simulink model "MRAC_PIDresp"  (R2018a)
settings: Solver=VariableStepAuto  StartTime=0.0  StopTime=100  RelTol=1e-3
values from neighbouring files (symbols this model uses):
  gam_p = 5    [MRAC_test.m]
  gam_pcmd = .1    (= 0.1)    [MRAC_test.m]
  k_d = 0.00073    [MRAC_test.m]
  k_i = 0    [MRAC_test.m]
  k_p = 0.0038    [MRAC_test.m]
  ref_den = [coef_a coef_b coef_c]    [MRAC_test.m]
  ref_num = [coef_c]    [MRAC_test.m]
libraries: simulink_extras x1
settings Model: Creator=ctf365  LastModifiedBy=ctf365

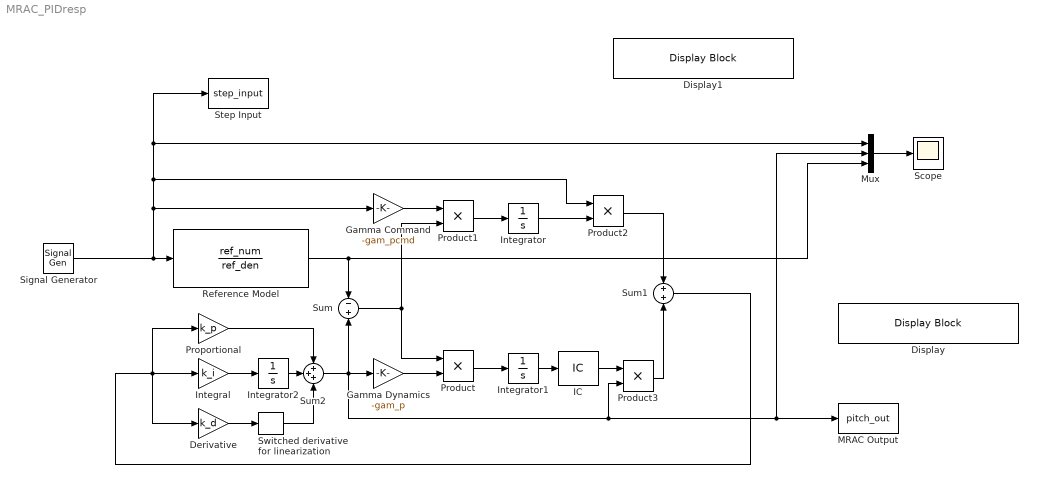
== system MRAC_PIDresp ==
  Derivative : Gain  Gain=k_d
  Display : DisplayBlock  WebBlockId=30  LabelPosition=Hide
  Display1 : DisplayBlock  WebBlockId=31  LabelPosition=Hide
  Gamma Command : Gain  Gain=-gam_pcmd
  Gamma Dynamics : Gain  Gain=-gam_p
  IC : InitialCondition  Value=-1.13
  Integral : Gain  Gain=k_i
  Integrator : Integrator
  Integrator1 : Integrator
  Integrator2 : Integrator
  MRAC Output : ToWorkspace  VariableName=pitch_out  SaveFormat=Timeseries  SampleTime=-1
  Mux : Mux  Inputs=3
  Product{,1..3} (4 alike) : Product
  Proportional : Gain  Gain=k_p
  Reference Model : TransferFcn  Numerator=ref_num  Denominator=ref_den
  Scope : Scope
  Signal Generator : SignalGenerator  WaveForm=square  Amplitude=20  Frequency=.2
  Step Input : ToWorkspace  VariableName=step_input  SaveFormat=Timeseries  SampleTime=-1
  Sum : Sum  Inputs=-+
  Sum1 : Sum
  Sum2 : Sum  Inputs=+++
  Switched derivative for linearization : simulink_extras/Linearization/Switched derivative for linearization  switchVal=1  derivConst=100
      settings: SourceProductName=Simulink  SourceProductBaseCode=SL
  wires:
  Signal Generator/1 -> Mux/1, Step Input/1, Product2/1, Gamma Command/1, Reference Model/1
  Reference Model/1 -> Mux/3, Sum/1
  Sum/1 -> Product/1, Product1/2
  Gamma Dynamics/1 -> Product/2
  Gamma Command/1 -> Product1/1
  Product/1 -> Integrator1/1
  Product1/1 -> Integrator/1
  Integrator/1 -> Product2/2
  Sum2/1 -> Sum/2, Gamma Dynamics/1, Product3/2, Mux/2, MRAC Output/1
  Integrator1/1 -> IC/1
  Product2/1 -> Sum1/1
  Product3/1 -> Sum1/2
  Sum1/1 -> Derivative/1, Proportional/1, Integral/1
  Integrator2/1 -> Sum2/2
  Proportional/1 -> Sum2/1
  Integral/1 -> Integrator2/1
  Derivative/1 -> Switched derivative for linearization/1
  Switched derivative for linearization/1 -> Sum2/3
  Mux/1 -> Scope/1
  IC/1 -> Product3/1
